simulink model "Off_Grid_Inverter_Control_LC"  (R2023b)
settings: Solver=FixedStepAuto  StartTime=0.0  StopTime=5  RelTol=1e-3
InitFcn:
  | %Initialization_for_Off_Grid_Inverter_Control_LC;
  | Initialization_for_Off_Grid_Inverter_Control_LC;
values from neighbouring files (symbols this model uses):
  C_grid = 45e-6    (= 4.5e-05)    [Initialization_for_Off_Grid_Inverter_Control_LC.m]
  Fnom_Grid = 50    [Initialization_for_Off_Grid_Inverter_Control_LC.m]
  Inom = Pnom/sqrt(3)/Unom_Grid    [Initialization_for_Off_Grid_Inverter_Control_LC.m]
  Ki_Idq = Kp_Idq*2*pi*0.5    (= 6.3165468167)    [Initialization_for_Off_Grid_Inverter_Control_LC.m]
  Ki_Phase = 10    [Initialization_for_Off_Grid_Inverter_Control_LC.m]
  Kp_Idq = L_grid*2*pi*1600    (= 2.0106192983)    [Initialization_for_Off_Grid_Inverter_Control_LC.m]
  Kp_Phase = 0.21    [Initialization_for_Off_Grid_Inverter_Control_LC.m]
  L_grid = 200e-6    (= 0.0002)    [Initialization_for_Off_Grid_Inverter_Control_LC.m]
  R_damping = 50    [Initialization_for_Off_Grid_Inverter_Control_LC.m]
  Ts_Control = 62.5e-6    (= 6.25e-05)    [Initialization_for_Off_Grid_Inverter_Control_LC.m]
  Udc_ref = 1500    [Initialization_for_Off_Grid_Inverter_Control_LC.m]
  Unom_Phase = Unom_Grid/sqrt(3)    [Initialization_for_Off_Grid_Inverter_Control_LC.m]
libraries: LibraryForCodeGeneration x19
settings Model: DataDictionary=Off_Grid_Inverter_Control_LC.sldd  Creator=ZZY  LastModifiedBy=ZZY
settings DataIOCC: ReturnWorkspaceOutputs=off
settings OptimizationCC: BlockReduction=off  DefaultParameterBehavior=Inlined  UseDivisionForNetSlopeComputation=on  DefaultUnderspecifiedDataType=single  ReuseModelBlockBuffer=off  ExpressionFolding=off  PassReuseOutputArgsAs=Individual arguments  ZeroExternalMemoryAtStartup=off  ZeroInternalMemoryAtStartup=off  EfficientFloat2IntCast=on  LifeSpan=inf  OptimizationLevel=level1  LabelGuidedReuse=on  EfficientTunableParamExpr=on
settings DebuggingCC: SignalInfNanChecking=warning  ReadBeforeWriteMsg=EnableAllAsError  WriteAfterWriteMsg=EnableAllAsError  WriteAfterReadMsg=EnableAllAsError  IntegerOverflowMsg=error  ParameterPrecisionLossMsg=none  ParameterTunabilityLossMsg=error  UniqueDataStoreMsg=error  AssertControl=DisableAll  NonBusSignalsTreatedAsBus=error  SFInvalidInputDataAccessInChartInitDiag=error  SFTransitionOutsideNaturalParentDiag=error  SFUnreachableExecutionPathDiag=error  SFUndirectedBroadcastEventsDiag=error  IntegerSaturationMsg=error
settings HardwareCC: ProdBitPerChar=16  ProdBitPerInt=16  ProdBitPerPointer=32  ProdBitPerSizeT=32  ProdBitPerPtrDiffT=32  ProdLargestAtomicInteger=Integer  ProdLargestAtomicFloat=None  ProdWordSize=16  ProdHWDeviceType=Texas Instruments->C2000  HardwareBoardFeatureSet=SoCBlockset
settings ModelReferenceCC: ModelReferenceNumInstancesAllowed=Single
settings SFSimCC: CompileTimeRecursionLimit=0  EnableRuntimeRecursion=off  MATLABDynamicMemAlloc=off
settings RTWCC: Description=Embedded Coder  SystemTargetFile=ert.tlc  TemplateMakefile=ert_default_tmf  GenerateReport=on  IncludeHyperlinkInReport=on  LaunchReport=on  DataTypeReplacement=CDataTypesFixedWidth  GenerateTraceInfo=on  GenerateTraceReport=on  GenerateTraceReportSl=on  GenerateTraceReportSf=on  GenerateTraceReportEml=on  GenerateWebview=on  GenerateCodeReplacementReport=on
settings CodeAppCC: ForceParamTrailComments=on  IgnoreCustomStorageClasses=off  OperatorAnnotations=on  SimulinkDataObjDesc=on  SFDataObjDesc=on  MATLABFcnDesc=on  InsertBlockDesc=on  StateflowObjectComments=on  MATLABSourceComments=on  EnableCustomComments=on  InlinedPrmAccess=Macros  ReqsInCode=on
settings ERTTargetCC: GenerateSampleERTMain=on  SupportNonFinite=off  ParenthesesLevel=Standards  CastingMode=Standards  GenerateSharedConstants=off  InlinedParameterPlacement=NonHierarchical  ERTCustomFileTemplate=example_file_process.tlc  RateTransitionBlockCode=Function  PreserveIfCondition=on  ConvertIfToSwitch=off  SuppressUnreachableDefaultCases=off  EnableSignedLeftShifts=off  EnableSignedRightShifts=off  MaxIdInt64=INT64_MAX  MinIdInt64=INT64_MIN  MaxIdUint64=UINT64_MAX  MaxIdInt32=INT32_MAX  MinIdInt32=INT32_MIN  MaxIdUint32=UINT32_MAX  MaxIdInt16=INT16_MAX  MinIdInt16=INT16_MIN  MaxIdUint16=UINT16_MAX  MaxIdInt8=INT8_MAX  MinIdInt8=INT8_MIN  MaxIdUint8=UINT8_MAX

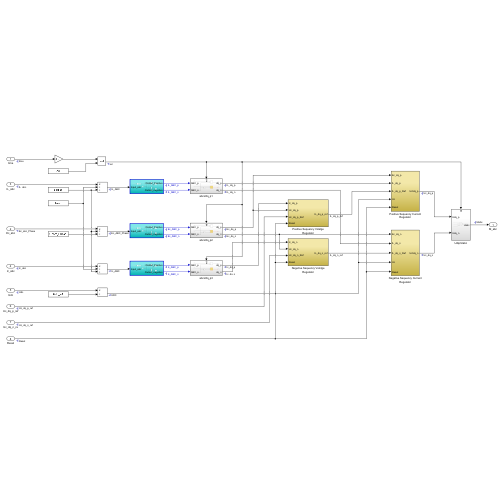
[thumbnail: Simulink's stored preview of the top-level diagram]
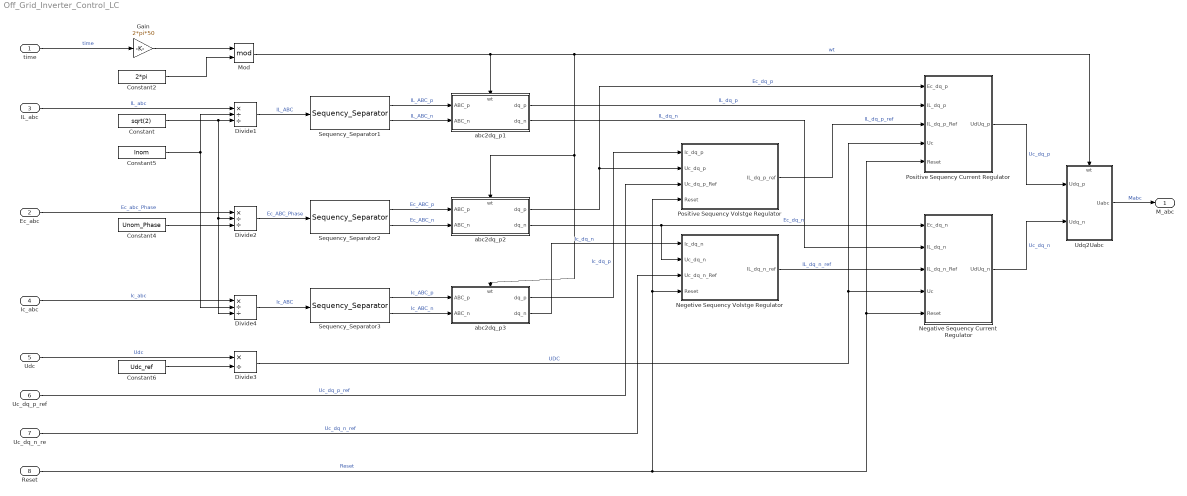
== system Off_Grid_Inverter_Control_LC ==
  time : Inport  OutDataTypeStr=single
  Ec_abc : Inport  Port=2
  IL_abc : Inport  Port=3  OutDataTypeStr=single
  Ic_abc : Inport  Port=4  OutDataTypeStr=single
  Udc : Inport  Port=5  OutDataTypeStr=single
  Uc_dq_p_ref : Inport  Port=6  OutDataTypeStr=single
  Uc_dq_n_re : Inport  Port=7  OutDataTypeStr=single
  Reset : Inport  Port=8  OutDataTypeStr=boolean
  Constant : Constant  Value=sqrt(2)  OutDataTypeStr=single  SampleTime=-1
  Constant2 : Constant  Value=2*pi  OutDataTypeStr=single  SampleTime=-1
  Constant4 : Constant  Value=Unom_Phase  OutDataTypeStr=Inherit: Inherit via back propagation  SampleTime=-1
  Constant5 : Constant  Value=Inom  OutDataTypeStr=Inherit: Inherit via back propagation  SampleTime=-1
  Constant6 : Constant  Value=Udc_ref  OutDataTypeStr=Inherit: Inherit via back propagation  SampleTime=-1
  Divide1 : Product  Inputs=*//  OutDataTypeStr=single
  Divide2 : Product  Inputs=*//  OutDataTypeStr=single
  Divide3 : Product  Inputs=*/  OutDataTypeStr=single
  Divide4 : Product  Inputs=*//  OutDataTypeStr=single
  Gain : Gain  Gain=2*pi*50
  Mod : Math  Operator=mod
  Negative Sequency Current Regulator : Subsystem
  Negetive Sequency Volstge Regulator : Subsystem
  Positive Sequency Current Regulator : Subsystem
  Positive Sequency Volstge Regulator : Subsystem
  Sequency_Separator1 : LibraryForCodeGeneration/Sequency_Separator  SystemSampleTime=-1  VariantActivationTime=update diagram  AllowFlexibleInterface=on  Latency=0  AutoFrameSizeCalculation=off
  Sequency_Separator2 : LibraryForCodeGeneration/Sequency_Separator  SystemSampleTime=-1  VariantActivationTime=update diagram  AllowFlexibleInterface=on  Latency=0  AutoFrameSizeCalculation=off
  Sequency_Separator3 : LibraryForCodeGeneration/Sequency_Separator  SystemSampleTime=-1  VariantActivationTime=update diagram  AllowFlexibleInterface=on  Latency=0  AutoFrameSizeCalculation=off
  Udq2Uabc : Subsystem
      settings: PortSchema="{\"entries\":[{\"content\":{\"sides\":[{\"content\":{\"connectorIds\":[\"In1\",\"In2\"]},\"type\":\"ConnectorPlacement.EquallySpacedRectSide\",\"uuid\":\"009786f4-728c-4160-b9bf-eaf0b5a05101\"},{\"content\":{\"connectorIds\":[\"Out1\"],\"side\":\"RIGHT\"},\"type\":\"ConnectorPlacement.EquallySpacedRectSide\",\"uuid\":\"2a94367a-5c57-4632-9573-ab089470159a\"},{\"content\":{\"connectorIds\":[\"In3\"],\"side\":\"TOP\"},\"type\":\"ConnectorPlacement.EquallySpacedRectSide\",\"uuid\":\"6906365b-3187-4c4b-97cf-c9dec4c5ef7c\"}]},\"type\":\"ConnectorPlacement.EquallySpacedConnector\",\"uuid\":\"96ca8566-a266-405c-817a-b47b433d51ed\"}],\"packageUris\":[\"http://schema.mathworks.com/mf0/Connector/R2020b\"],\"version\":\"1.0\"}"
  abc2dq_p1 : Subsystem
      settings: PortSchema="{\"entries\":[{\"content\":{\"sides\":[{\"content\":{\"connectorIds\":[\"In1\",\"In2\"]},\"type\":\"ConnectorPlacement.EquallySpacedRectSide\",\"uuid\":\"702c7fae-dbbb-427d-af19-afd468018ae6\"},{\"content\":{\"connectorIds\":[\"Out1\",\"Out2\"],\"side\":\"RIGHT\"},\"type\":\"ConnectorPlacement.EquallySpacedRectSide\",\"uuid\":\"d2ca5462-a446-46d8-bb73-1a455ffa959f\"},{\"content\":{\"connectorIds\":[\"In3\"],\"side\":\"TOP\"},\"type\":\"ConnectorPlacement.EquallySpacedRectSide\",\"uuid\":\"50bc6c44-424f-4342-960e-11540364fe97\"}]},\"type\":\"ConnectorPlacement.EquallySpacedConnector\",\"uuid\":\"f58cf64d-fe35-43f1-a031-7ee625a8bb1e\"}],\"packageUris\":[\"http://schema.mathworks.com/mf0/Connector/R2020b\"],\"version\":\"1.0\"}"
  abc2dq_p2 : Subsystem
      settings: PortSchema="{\"entries\":[{\"content\":{\"sides\":[{\"content\":{\"connectorIds\":[\"In1\",\"In2\"]},\"type\":\"ConnectorPlacement.EquallySpacedRectSide\",\"uuid\":\"702c7fae-dbbb-427d-af19-afd468018ae6\"},{\"content\":{\"connectorIds\":[\"Out1\",\"Out2\"],\"side\":\"RIGHT\"},\"type\":\"ConnectorPlacement.EquallySpacedRectSide\",\"uuid\":\"d2ca5462-a446-46d8-bb73-1a455ffa959f\"},{\"content\":{\"connectorIds\":[\"In3\"],\"side\":\"TOP\"},\"type\":\"ConnectorPlacement.EquallySpacedRectSide\",\"uuid\":\"50bc6c44-424f-4342-960e-11540364fe97\"}]},\"type\":\"ConnectorPlacement.EquallySpacedConnector\",\"uuid\":\"f58cf64d-fe35-43f1-a031-7ee625a8bb1e\"}],\"packageUris\":[\"http://schema.mathworks.com/mf0/Connector/R2020b\"],\"version\":\"1.0\"}"
  abc2dq_p3 : Subsystem
      settings: PortSchema="{\"entries\":[{\"content\":{\"sides\":[{\"content\":{\"connectorIds\":[\"In1\",\"In2\"]},\"type\":\"ConnectorPlacement.EquallySpacedRectSide\",\"uuid\":\"702c7fae-dbbb-427d-af19-afd468018ae6\"},{\"content\":{\"connectorIds\":[\"Out1\",\"Out2\"],\"side\":\"RIGHT\"},\"type\":\"ConnectorPlacement.EquallySpacedRectSide\",\"uuid\":\"d2ca5462-a446-46d8-bb73-1a455ffa959f\"},{\"content\":{\"connectorIds\":[\"In3\"],\"side\":\"TOP\"},\"type\":\"ConnectorPlacement.EquallySpacedRectSide\",\"uuid\":\"50bc6c44-424f-4342-960e-11540364fe97\"}]},\"type\":\"ConnectorPlacement.EquallySpacedConnector\",\"uuid\":\"f58cf64d-fe35-43f1-a031-7ee625a8bb1e\"}],\"packageUris\":[\"http://schema.mathworks.com/mf0/Connector/R2020b\"],\"version\":\"1.0\"}"
  M_abc : Outport  OutDataTypeStr=single
  wires:
  Negative Sequency Current Regulator/1(UdUq_n) -> Udq2Uabc/2(Udq_n)  "Uc_dq_n"
  Constant/1 -> Divide2/2, Divide4/3, Divide1/3
  Sequency_Separator1/1 -> abc2dq_p1/1("ABC_p ")  "IL_ABC_p"
  Positive Sequency Volstge Regulator/1(IL_dq_p_ref) -> Positive Sequency Current Regulator/3(IL_dq_p_Ref)  "IL_dq_p_ref"
  abc2dq_p1/1(dq_p) -> Positive Sequency Current Regulator/2(IL_dq_p)  "IL_dq_p"
  Sequency_Separator3/2 -> abc2dq_p3/2("ABC_n ")  "Ic_ABC_n"
  abc2dq_p3/1(dq_p) -> Positive Sequency Volstge Regulator/1(Ic_dq_p)  "Ic_dq_p"
  Uc_dq_p_ref/1 -> Positive Sequency Volstge Regulator/3(Uc_dq_p_Ref)  "Uc_dq_p_ref"
  Sequency_Separator3/1 -> abc2dq_p3/1("ABC_p ")  "Ic_ABC_p"
  Ec_abc/1 -> Divide2/1  "Ec_abc_Phase"
  time/1 -> Gain/1  "time"
  abc2dq_p1/2(dq_n) -> Negative Sequency Current Regulator/2(IL_dq_n)  "IL_dq_n"
  abc2dq_p2/1(dq_p) -> Positive Sequency Volstge Regulator/2(Uc_dq_p), Positive Sequency Current Regulator/1(Ec_dq_p)  "Ec_dq_p"
  Divide3/1 -> Positive Sequency Current Regulator/4(Uc), Negative Sequency Current Regulator/4(Uc)  "UDC"
  Constant6/1 -> Divide3/2
  Sequency_Separator1/2 -> abc2dq_p1/2("ABC_n ")  "IL_ABC_n"
  abc2dq_p2/2(dq_n) -> Negetive Sequency Volstge Regulator/2(Uc_dq_n), Negative Sequency Current Regulator/1(Ec_dq_n)  "Ec_dq_n"
  Sequency_Separator2/1 -> abc2dq_p2/1("ABC_p ")  "Ec_ABC_p"
  Constant4/1 -> Divide2/3
  Ic_abc/1 -> Divide4/1  "Ic_abc"
  Negetive Sequency Volstge Regulator/1(IL_dq_n_ref) -> Negative Sequency Current Regulator/3(IL_dq_n_Ref)  "IL_dq_n_ref"
  Sequency_Separator2/2 -> abc2dq_p2/2("ABC_n ")  "Ec_ABC_n"
  Divide2/1 -> Sequency_Separator2/1  "Ec_ABC_Phase"
  Divide4/1 -> Sequency_Separator3/1  "Ic_ABC"
  Reset/1 -> Positive Sequency Volstge Regulator/4(Reset), Negetive Sequency Volstge Regulator/4(Reset), Positive Sequency Current Regulator/5(Reset), Negative Sequency Current Regulator/5(Reset)  "Reset"
  Constant5/1 -> Divide4/2, Divide1/2
  Positive Sequency Current Regulator/1(UdUq_p) -> Udq2Uabc/1(Udq_p)  "Uc_dq_p"
  IL_abc/1 -> Divide1/1  "IL_abc"
  Constant2/1 -> Mod/2
  Mod/1 -> Udq2Uabc/3(wt), abc2dq_p2/3(wt), abc2dq_p3/3(wt), abc2dq_p1/3(wt)  "wt"
  Udq2Uabc/1(Uabc) -> M_abc/1  "Mabc"
  Divide1/1 -> Sequency_Separator1/1  "IL_ABC"
  Udc/1 -> Divide3/1  "Udc"
  Gain/1 -> Mod/1
  abc2dq_p3/2(dq_n) -> Negetive Sequency Volstge Regulator/1(Ic_dq_n)  "Ic_dq_n"
  Uc_dq_n_re/1 -> Negetive Sequency Volstge Regulator/3(Uc_dq_n_Ref)  "Uc_dq_n_ref"

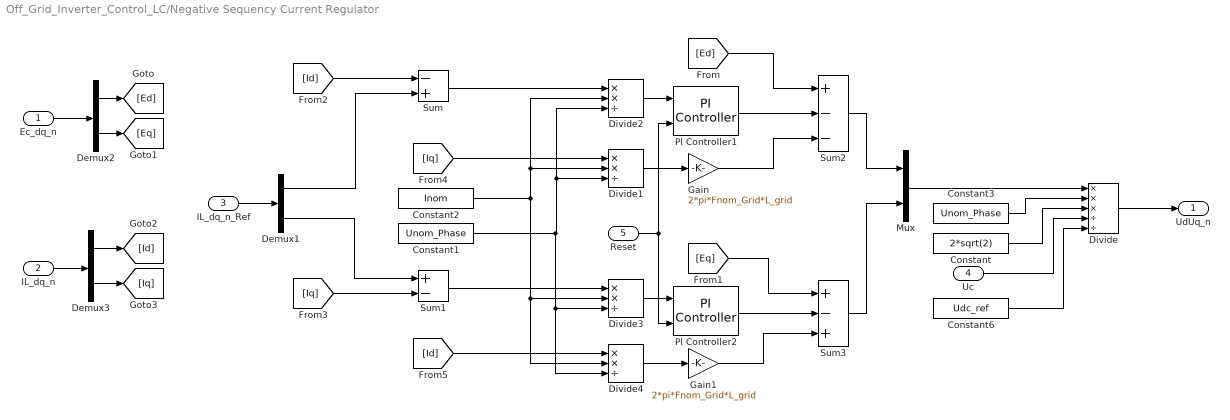
== system Off_Grid_Inverter_Control_LC/Negative Sequency Current Regulator ==
  Ec_dq_n : Inport
  IL_dq_n : Inport  Port=2
  IL_dq_n_Ref : Inport  Port=3
  Uc : Inport  Port=4
  Reset : Inport  Port=5  OutDataTypeStr=boolean
  Constant : Constant  Value=2*sqrt(2)  OutDataTypeStr=Inherit: Inherit via back propagation  SampleTime=-1
  Constant1 : Constant  Value=Unom_Phase  OutDataTypeStr=Inherit: Inherit via back propagation  SampleTime=-1
  Constant2 : Constant  Value=Inom  OutDataTypeStr=Inherit: Inherit via back propagation  SampleTime=-1
  Constant3 : Constant  Value=Unom_Phase  OutDataTypeStr=Inherit: Inherit via back propagation  SampleTime=-1
  Constant6 : Constant  Value=Udc_ref  OutDataTypeStr=Inherit: Inherit via back propagation  SampleTime=-1
  Demux1 : Demux  Outputs=2
  Demux2 : Demux  Outputs=2
  Demux3 : Demux  Outputs=2
  Divide : Product  Inputs=***//  OutDataTypeStr=single
  Divide{1..4} (4 alike) : Product  Inputs=**/  OutDataTypeStr=single
  Gain : Gain  Gain=2*pi*Fnom_Grid*L_grid  ParamDataTypeStr=Inherit: Same as input
  Gain1 : Gain  Gain=2*pi*Fnom_Grid*L_grid  ParamDataTypeStr=Inherit: Same as input
  Mux : Mux  Inputs=2
  PI Controller1 : LibraryForCodeGeneration/PI Controller  Kp=Kp_Idq  Ki=Ki_Idq  Ts=Ts_Control  Max=2  Min=-2
  PI Controller2 : LibraryForCodeGeneration/PI Controller  Kp=Kp_Idq  Ki=Ki_Idq  Ts=Ts_Control  Max=2  Min=-2
  Sum : Sum  Inputs=-+  InputSameDT=on  SaturateOnIntegerOverflow=on  OutDataTypeStr=Inherit: Same as first input
  Sum1 : Sum  Inputs=+-  InputSameDT=on  SaturateOnIntegerOverflow=on  OutDataTypeStr=Inherit: Same as first input
  Sum2 : Sum  Inputs=+--  InputSameDT=on  SaturateOnIntegerOverflow=on  OutDataTypeStr=Inherit: Same as first input
  Sum3 : Sum  Inputs=+-+  InputSameDT=on  SaturateOnIntegerOverflow=on  OutDataTypeStr=Inherit: Same as first input
  UdUq_n : Outport
  wires:
  [Id] -> Divide4/1
  [Iq] -> Divide1/1
  [Iq] -> Sum1/2
  [Id] -> Sum/1
  IL_dq_n/1 -> Demux3/1
  Demux3/1 -> [Id]
  Demux3/2 -> [Iq]
  Demux1/2 -> Sum1/1
  Demux1/1 -> Sum/2
  [Eq] -> Sum3/1
  [Ed] -> Sum2/1
  Demux2/2 -> [Eq]
  Demux2/1 -> [Ed]
  Divide3/1 -> PI Controller2/1
  Sum/1 -> Divide2/1
  Mux/1 -> Divide/1
  Divide/1 -> UdUq_n/1
  Gain1/1 -> Sum3/3
  Gain/1 -> Sum2/3
  Ec_dq_n/1 -> Demux2/1
  IL_dq_n_Ref/1 -> Demux1/1
  Sum2/1 -> Mux/1
  Sum1/1 -> Divide3/1
  Divide2/1 -> PI Controller1/1
  Sum3/1 -> Mux/2
  Reset/1 -> PI Controller1/2, PI Controller2/2
  Constant3/1 -> Divide/2
  Constant/1 -> Divide/3
  Uc/1 -> Divide/4
  Constant6/1 -> Divide/5
  Divide1/1 -> Gain/1
  Divide4/1 -> Gain1/1
  Constant2/1 -> Divide1/2, Divide2/2, Divide4/2, Divide3/2
  Constant1/1 -> Divide3/3, Divide4/3, Divide1/3, Divide2/3
  PI Controller2/1 -> Sum3/2
  PI Controller1/1 -> Sum2/2

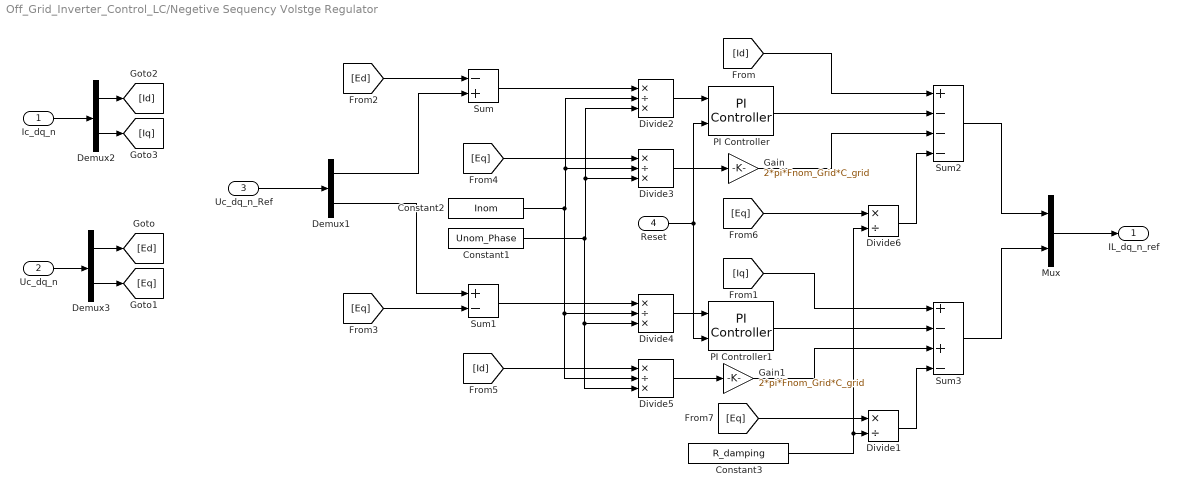
== system Off_Grid_Inverter_Control_LC/Negetive Sequency Volstge Regulator ==
  Ic_dq_n : Inport
  Uc_dq_n : Inport  Port=2
  Uc_dq_n_Ref : Inport  Port=3
  Reset : Inport  Port=4  OutDataTypeStr=boolean
  Constant1 : Constant  Value=Unom_Phase  OutDataTypeStr=Inherit: Inherit via back propagation  SampleTime=-1
  Constant2 : Constant  Value=Inom  OutDataTypeStr=Inherit: Inherit via back propagation  SampleTime=-1
  Constant3 : Constant  Value=R_damping  OutDataTypeStr=Inherit: Inherit via back propagation  SampleTime=-1
  Demux1 : Demux  Outputs=2
  Demux2 : Demux  Outputs=2
  Demux3 : Demux  Outputs=2
  Divide1 : Product  Inputs=*/
  Divide{2..5} (4 alike) : Product  Inputs=*/*  OutDataTypeStr=single
  Divide6 : Product  Inputs=*/
  Gain : Gain  Gain=2*pi*Fnom_Grid*C_grid  ParamDataTypeStr=Inherit: Same as input
  Gain1 : Gain  Gain=2*pi*Fnom_Grid*C_grid  ParamDataTypeStr=Inherit: Same as input
  Mux : Mux  Inputs=2
  PI Controller : LibraryForCodeGeneration/PI Controller  Kp=Kp_Phase  Ki=Ki_Phase  Ts=Ts_Control  Max=2  Min=-2
  PI Controller1 : LibraryForCodeGeneration/PI Controller  Kp=Kp_Phase  Ki=Ki_Phase  Ts=Ts_Control  Max=2  Min=-2
  Sum : Sum  Inputs=-+  InputSameDT=on  SaturateOnIntegerOverflow=on  OutDataTypeStr=Inherit: Same as first input
  Sum1 : Sum  Inputs=+-  InputSameDT=on  SaturateOnIntegerOverflow=on  OutDataTypeStr=Inherit: Same as first input
  Sum2 : Sum  Inputs=+---  InputSameDT=on  SaturateOnIntegerOverflow=on  OutDataTypeStr=Inherit: Same as first input
  Sum3 : Sum  Inputs=+-+-  InputSameDT=on  SaturateOnIntegerOverflow=on  OutDataTypeStr=Inherit: Same as first input
  IL_dq_n_ref : Outport
  wires:
  Sum3/1 -> Mux/2
  Sum1/1 -> Divide4/1
  Sum2/1 -> Mux/1
  Uc_dq_n_Ref/1 -> Demux1/1
  Divide3/1 -> Gain/1
  Divide5/1 -> Gain1/1
  Ic_dq_n/1 -> Demux2/1
  Gain/1 -> Sum2/3
  Mux/1 -> IL_dq_n_ref/1
  Sum/1 -> Divide2/1
  Divide4/1 -> PI Controller1/1
  Demux2/1 -> [Id]
  Demux2/2 -> [Iq]
  [Id] -> Sum2/1
  Demux1/1 -> Sum/2
  Demux1/2 -> Sum1/1
  Demux3/2 -> [Eq]
  Demux3/1 -> [Ed]
  Uc_dq_n/1 -> Demux3/1
  [Ed] -> Sum/1
  [Eq] -> Sum1/2
  [Eq] -> Divide3/1
  [Id] -> Divide5/1
  PI Controller/1 -> Sum2/2
  Divide2/1 -> PI Controller/1
  Reset/1 -> PI Controller1/2, PI Controller/2
  Constant2/1 -> Divide5/2, Divide4/2, Divide3/2, Divide2/2
  Constant1/1 -> Divide5/3, Divide4/3, Divide3/3, Divide2/3
  [Iq] -> Sum3/1
  PI Controller1/1 -> Sum3/2
  Gain1/1 -> Sum3/3
  [Eq] -> Divide1/1
  Divide1/1 -> Sum3/4
  [Eq] -> Divide6/1
  Constant3/1 -> Divide6/2, Divide1/2
  Divide6/1 -> Sum2/4

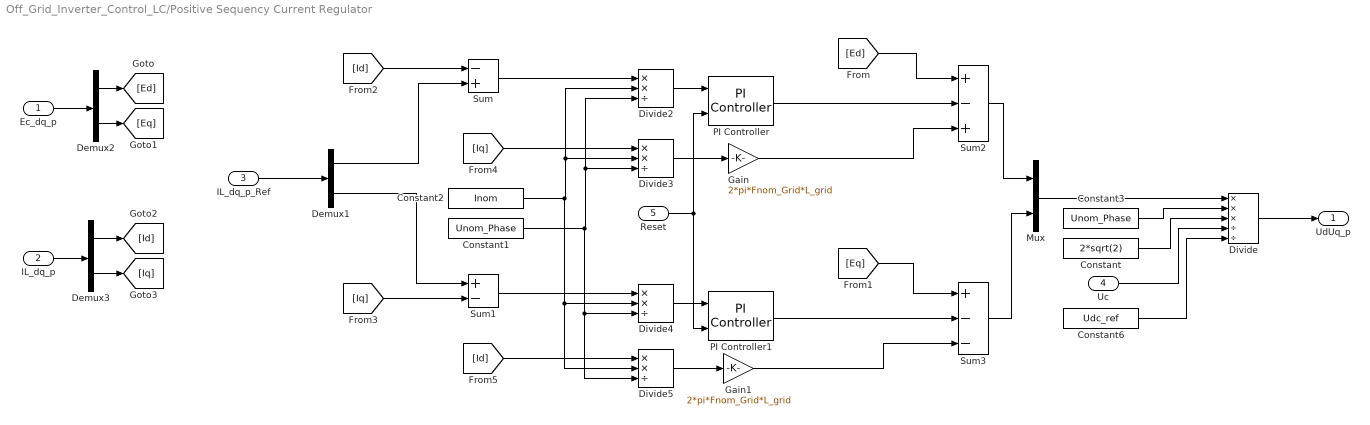
== system Off_Grid_Inverter_Control_LC/Positive Sequency Current Regulator ==
  Ec_dq_p : Inport
  IL_dq_p : Inport  Port=2
  IL_dq_p_Ref : Inport  Port=3
  Uc : Inport  Port=4
  Reset : Inport  Port=5  OutDataTypeStr=boolean
  Constant : Constant  Value=2*sqrt(2)  OutDataTypeStr=Inherit: Inherit via back propagation  SampleTime=-1
  Constant1 : Constant  Value=Unom_Phase  OutDataTypeStr=Inherit: Inherit via back propagation  SampleTime=-1
  Constant2 : Constant  Value=Inom  OutDataTypeStr=Inherit: Inherit via back propagation  SampleTime=-1
  Constant3 : Constant  Value=Unom_Phase  OutDataTypeStr=Inherit: Inherit via back propagation  SampleTime=-1
  Constant6 : Constant  Value=Udc_ref  OutDataTypeStr=Inherit: Inherit via back propagation  SampleTime=-1
  Demux1 : Demux  Outputs=2
  Demux2 : Demux  Outputs=2
  Demux3 : Demux  Outputs=2
  Divide : Product  Inputs=***//  OutDataTypeStr=single
  Divide{2..5} (4 alike) : Product  Inputs=**/  OutDataTypeStr=single
  Gain : Gain  Gain=2*pi*Fnom_Grid*L_grid  ParamDataTypeStr=Inherit: Same as input
  Gain1 : Gain  Gain=2*pi*Fnom_Grid*L_grid  ParamDataTypeStr=Inherit: Same as input
  Mux : Mux  Inputs=2
  PI Controller : LibraryForCodeGeneration/PI Controller  Kp=Kp_Idq  Ki=Ki_Idq  Ts=Ts_Control  Max=2  Min=-2
  PI Controller1 : LibraryForCodeGeneration/PI Controller  Kp=Kp_Idq  Ki=Ki_Idq  Ts=Ts_Control  Max=2  Min=-2
  Sum : Sum  Inputs=-+  InputSameDT=on  SaturateOnIntegerOverflow=on  OutDataTypeStr=Inherit: Same as first input
  Sum1 : Sum  Inputs=+-  InputSameDT=on  SaturateOnIntegerOverflow=on  OutDataTypeStr=Inherit: Same as first input
  Sum2 : Sum  Inputs=+-+  InputSameDT=on  SaturateOnIntegerOverflow=on  OutDataTypeStr=Inherit: Same as first input
  Sum3 : Sum  Inputs=+--  InputSameDT=on  SaturateOnIntegerOverflow=on  OutDataTypeStr=Inherit: Same as first input
  UdUq_p : Outport
  wires:
  Sum3/1 -> Mux/2
  Sum2/1 -> Mux/1
  IL_dq_p_Ref/1 -> Demux1/1
  Uc/1 -> Divide/4
  Divide3/1 -> Gain/1
  Divide5/1 -> Gain1/1
  Ec_dq_p/1 -> Demux2/1
  Gain/1 -> Sum2/3
  Divide/1 -> UdUq_p/1
  Mux/1 -> Divide/1
  Sum/1 -> Divide2/1
  Divide4/1 -> PI Controller1/1
  Demux2/1 -> [Ed]
  Demux2/2 -> [Eq]
  [Ed] -> Sum2/1
  Demux1/1 -> Sum/2
  Demux1/2 -> Sum1/1
  Demux3/2 -> [Iq]
  Demux3/1 -> [Id]
  IL_dq_p/1 -> Demux3/1
  [Id] -> Sum/1
  [Iq] -> Sum1/2
  [Iq] -> Divide3/1
  [Id] -> Divide5/1
  Divide2/1 -> PI Controller/1
  Reset/1 -> PI Controller1/2, PI Controller/2
  Constant3/1 -> Divide/2
  Constant/1 -> Divide/3
  Constant6/1 -> Divide/5
  Constant2/1 -> Divide5/2, Divide4/2, Divide3/2, Divide2/2
  Constant1/1 -> Divide5/3, Divide4/3, Divide3/3, Divide2/3
  [Eq] -> Sum3/1
  Gain1/1 -> Sum3/3
  PI Controller1/1 -> Sum3/2
  Sum1/1 -> Divide4/1
  PI Controller/1 -> Sum2/2

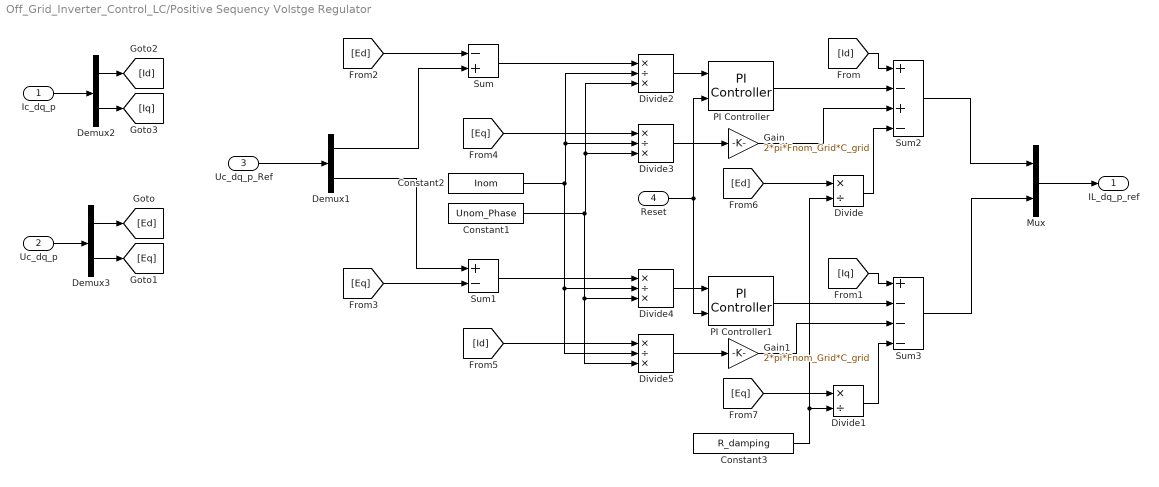
== system Off_Grid_Inverter_Control_LC/Positive Sequency Volstge Regulator ==
  Ic_dq_p : Inport
  Uc_dq_p : Inport  Port=2
  Uc_dq_p_Ref : Inport  Port=3
  Reset : Inport  Port=4  OutDataTypeStr=boolean
  Constant1 : Constant  Value=Unom_Phase  OutDataTypeStr=Inherit: Inherit via back propagation  SampleTime=-1
  Constant2 : Constant  Value=Inom  OutDataTypeStr=Inherit: Inherit via back propagation  SampleTime=-1
  Constant3 : Constant  Value=R_damping  OutDataTypeStr=Inherit: Inherit via back propagation  SampleTime=-1
  Demux1 : Demux  Outputs=2
  Demux2 : Demux  Outputs=2
  Demux3 : Demux  Outputs=2
  Divide : Product  Inputs=*/
  Divide1 : Product  Inputs=*/
  Divide{2..5} (4 alike) : Product  Inputs=*/*  OutDataTypeStr=single
  Gain : Gain  Gain=2*pi*Fnom_Grid*C_grid  ParamDataTypeStr=Inherit: Same as input
  Gain1 : Gain  Gain=2*pi*Fnom_Grid*C_grid  ParamDataTypeStr=Inherit: Same as input
  Mux : Mux  Inputs=2
  PI Controller : LibraryForCodeGeneration/PI Controller  Kp=Kp_Phase  Ki=Ki_Phase  Ts=Ts_Control  Max=2  Min=-2
  PI Controller1 : LibraryForCodeGeneration/PI Controller  Kp=Kp_Phase  Ki=Ki_Phase  Ts=Ts_Control  Max=2  Min=-2
  Sum : Sum  Inputs=-+  InputSameDT=on  SaturateOnIntegerOverflow=on  OutDataTypeStr=Inherit: Same as first input
  Sum1 : Sum  Inputs=+-  InputSameDT=on  SaturateOnIntegerOverflow=on  OutDataTypeStr=Inherit: Same as first input
  Sum2 : Sum  Inputs=+-+-  InputSameDT=on  SaturateOnIntegerOverflow=on  OutDataTypeStr=Inherit: Same as first input
  Sum3 : Sum  Inputs=+---  InputSameDT=on  SaturateOnIntegerOverflow=on  OutDataTypeStr=Inherit: Same as first input
  IL_dq_p_ref : Outport
  wires:
  Sum3/1 -> Mux/2
  Sum1/1 -> Divide4/1
  Sum2/1 -> Mux/1
  Uc_dq_p_Ref/1 -> Demux1/1
  Divide3/1 -> Gain/1
  Divide5/1 -> Gain1/1
  Ic_dq_p/1 -> Demux2/1
  Gain/1 -> Sum2/3
  Mux/1 -> IL_dq_p_ref/1
  Sum/1 -> Divide2/1
  Divide4/1 -> PI Controller1/1
  Demux2/1 -> [Id]
  Demux2/2 -> [Iq]
  [Id] -> Sum2/1
  Demux1/1 -> Sum/2
  Demux1/2 -> Sum1/1
  Demux3/2 -> [Eq]
  Demux3/1 -> [Ed]
  Uc_dq_p/1 -> Demux3/1
  [Ed] -> Sum/1
  [Eq] -> Sum1/2
  [Eq] -> Divide3/1
  [Id] -> Divide5/1
  PI Controller/1 -> Sum2/2
  Divide2/1 -> PI Controller/1
  Reset/1 -> PI Controller1/2, PI Controller/2
  Constant2/1 -> Divide5/2, Divide4/2, Divide3/2, Divide2/2
  Constant1/1 -> Divide5/3, Divide4/3, Divide3/3, Divide2/3
  [Iq] -> Sum3/1
  PI Controller1/1 -> Sum3/2
  Gain1/1 -> Sum3/3
  [Ed] -> Divide/1
  Divide/1 -> Sum2/4
  Divide1/1 -> Sum3/4
  [Eq] -> Divide1/1
  Constant3/1 -> Divide1/2, Divide/2

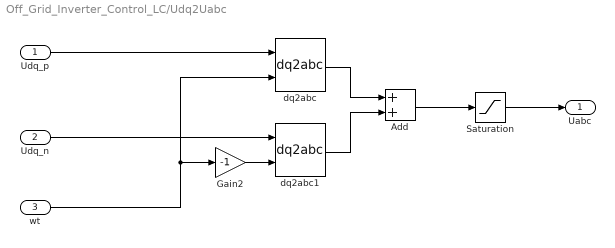
== system Off_Grid_Inverter_Control_LC/Udq2Uabc ==
  Udq_p : Inport
  Udq_n : Inport  Port=2
  wt : Inport  Port=3
  Add : Sum
  Gain2 : Gain  Gain=-1  ParamDataTypeStr=Inherit: Same as input
  Saturation : Saturate  UpperLimit=1.15  LowerLimit=-1.15
  dq2abc : LibraryForCodeGeneration/dq2abc  SystemSampleTime=-1  VariantActivationTime=update diagram  AllowFlexibleInterface=on  Latency=0  AutoFrameSizeCalculation=off
  dq2abc1 : LibraryForCodeGeneration/dq2abc  SystemSampleTime=-1  VariantActivationTime=update diagram  AllowFlexibleInterface=on  Latency=0  AutoFrameSizeCalculation=off
  Uabc : Outport
  wires:
  dq2abc1/1 -> Add/2
  wt/1 -> dq2abc/2, Gain2/1
  Gain2/1 -> dq2abc1/2
  Udq_p/1 -> dq2abc/1
  Udq_n/1 -> dq2abc1/1
  Add/1 -> Saturation/1
  dq2abc/1 -> Add/1
  Saturation/1 -> Uabc/1

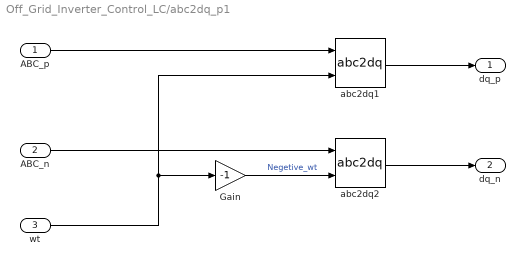
== system Off_Grid_Inverter_Control_LC/abc2dq_p1 ==
  "ABC_p " : Inport
  "ABC_n " : Inport  Port=2
  wt : Inport  Port=3
  Gain : Gain  Gain=-1
  abc2dq1 : LibraryForCodeGeneration/abc2dq  SystemSampleTime=-1  VariantActivationTime=update diagram  AllowFlexibleInterface=on  Latency=0  AutoFrameSizeCalculation=off
  abc2dq2 : LibraryForCodeGeneration/abc2dq  SystemSampleTime=-1  VariantActivationTime=update diagram  AllowFlexibleInterface=on  Latency=0  AutoFrameSizeCalculation=off
  dq_p : Outport
  dq_n : Outport  Port=2
  wires:
  "ABC_p "/1 -> abc2dq1/1
  abc2dq1/1 -> dq_p/1
  Gain/1 -> abc2dq2/2  "Negetive_wt"
  "ABC_n "/1 -> abc2dq2/1
  abc2dq2/1 -> dq_n/1
  wt/1 -> abc2dq1/2, Gain/1

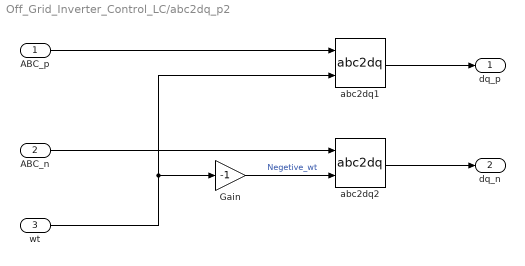
== system Off_Grid_Inverter_Control_LC/abc2dq_p2 ==
  "ABC_p " : Inport
  "ABC_n " : Inport  Port=2
  wt : Inport  Port=3
  Gain : Gain  Gain=-1
  abc2dq1 : LibraryForCodeGeneration/abc2dq  SystemSampleTime=-1  VariantActivationTime=update diagram  AllowFlexibleInterface=on  Latency=0  AutoFrameSizeCalculation=off
  abc2dq2 : LibraryForCodeGeneration/abc2dq  SystemSampleTime=-1  VariantActivationTime=update diagram  AllowFlexibleInterface=on  Latency=0  AutoFrameSizeCalculation=off
  dq_p : Outport
  dq_n : Outport  Port=2
  wires:
  "ABC_p "/1 -> abc2dq1/1
  abc2dq1/1 -> dq_p/1
  Gain/1 -> abc2dq2/2  "Negetive_wt"
  "ABC_n "/1 -> abc2dq2/1
  abc2dq2/1 -> dq_n/1
  wt/1 -> abc2dq1/2, Gain/1

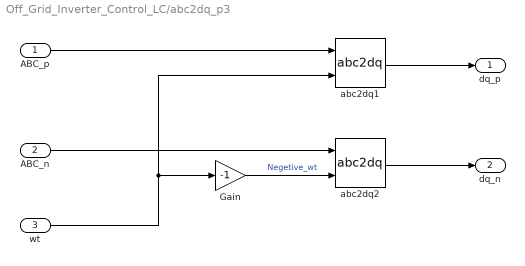
== system Off_Grid_Inverter_Control_LC/abc2dq_p3 ==
  "ABC_p " : Inport
  "ABC_n " : Inport  Port=2
  wt : Inport  Port=3
  Gain : Gain  Gain=-1
  abc2dq1 : LibraryForCodeGeneration/abc2dq  SystemSampleTime=-1  VariantActivationTime=update diagram  AllowFlexibleInterface=on  Latency=0  AutoFrameSizeCalculation=off
  abc2dq2 : LibraryForCodeGeneration/abc2dq  SystemSampleTime=-1  VariantActivationTime=update diagram  AllowFlexibleInterface=on  Latency=0  AutoFrameSizeCalculation=off
  dq_p : Outport
  dq_n : Outport  Port=2
  wires:
  "ABC_p "/1 -> abc2dq1/1
  abc2dq1/1 -> dq_p/1
  Gain/1 -> abc2dq2/2  "Negetive_wt"
  "ABC_n "/1 -> abc2dq2/1
  abc2dq2/1 -> dq_n/1
  wt/1 -> abc2dq1/2, Gain/1
